simulink model "GS_s_v_seno_function"  (R2023b)
settings: Solver=VariableStepAuto  StartTime=0.0  StopTime=50  RelTol=1e-7
values from neighbouring files (symbols this model uses):
  omega_n = 2.63/Tr    (= 9.74074074074)    [gain_sheduling_WP5.m]
  zita = input(2)    [GS_compute_gains_PP.m]    (also in compute_gains_WP5.m; gain_sheduling_WP5.m = 0.95)
undefined symbols (not defined in the file or in its folder): LQR_activate
settings Model: Creator=miche  LastModifiedBy=miche

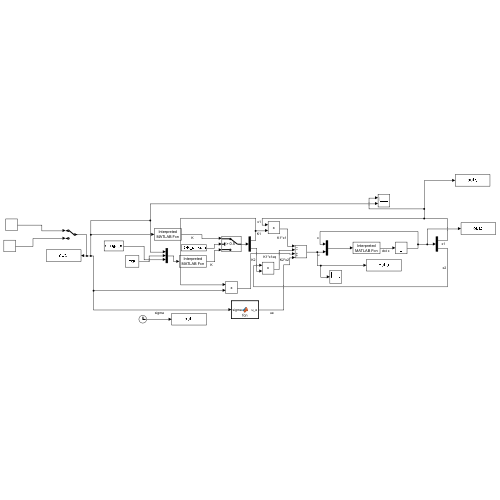
[thumbnail: Simulink's stored preview of the top-level diagram]
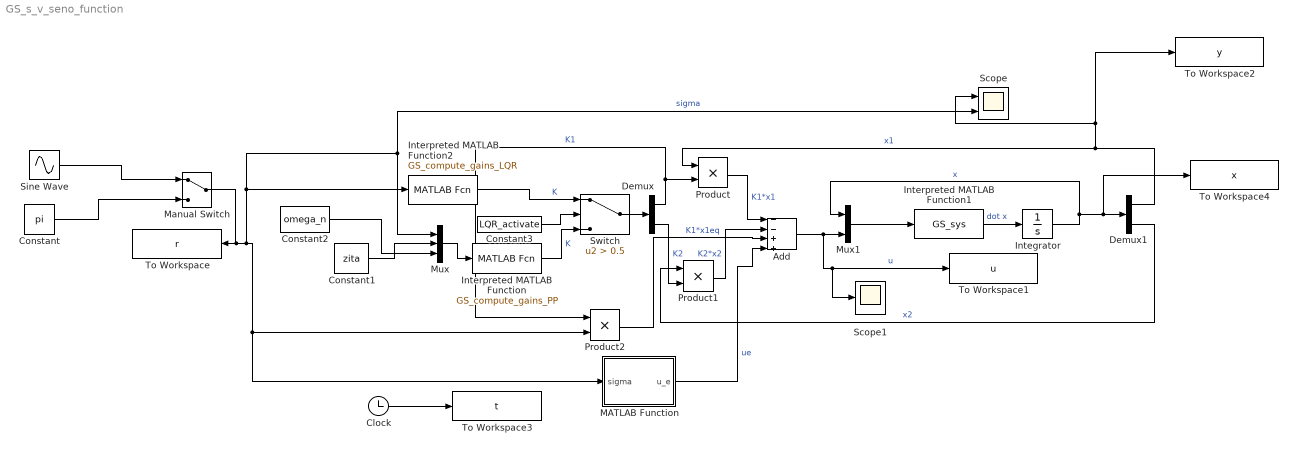
== system GS_s_v_seno_function ==
  Add : Sum  Inputs=--++
  Clock : Clock
  Constant : Constant  Value=pi
  Constant1 : Constant  Value=zita
  Constant2 : Constant  Value=omega_n
  Constant3 : Constant  Value=LQR_activate
  Demux : Demux  Outputs=2
  Demux1 : Demux  Outputs=2
  Integrator : Integrator
  Interpreted MATLAB Function : MATLABFcn  MATLABFcn=GS_compute_gains_PP  OutputDimensions=2
  Interpreted MATLAB Function1 : MATLABFcn  MATLABFcn=GS_sys  OutputDimensions=2
  Interpreted MATLAB Function2 : MATLABFcn  MATLABFcn=GS_compute_gains_LQR  OutputDimensions=2
  MATLAB Function : MATLAB Function  TreatAsAtomicUnit=on
  Manual Switch : ManualSwitch
  Mux : Mux  Inputs=3
  Mux1 : Mux  Inputs=2
  Product : Product
  Product1 : Product
  Product2 : Product
  Scope : Scope  NumInputPorts=2
  Scope1 : Scope
  Sine Wave : Sin  Amplitude=3.14  SampleTime=0
  Switch : Switch  Criteria=u2 > Threshold  Threshold=0.5  SaturateOnIntegerOverflow=off  InputSameDT=off
  To Workspace : ToWorkspace  VariableName=r  SampleTime=-1
  To Workspace1 : ToWorkspace  VariableName=u  SampleTime=-1
  To Workspace2 : ToWorkspace  VariableName=y  SampleTime=-1
  To Workspace3 : ToWorkspace  VariableName=t  SampleTime=-1
  To Workspace4 : ToWorkspace  VariableName=x  SampleTime=-1
  wires:
  Mux/1 -> Interpreted MATLAB Function/1
  Constant/1 -> Manual Switch/2
  Manual Switch/1 -> Scope/2, Mux/1, Interpreted MATLAB Function2/1, MATLAB Function/1(sigma), Product2/2, To Workspace/1  "sigma"
  Mux1/1 -> Interpreted MATLAB Function1/1
  Interpreted MATLAB Function1/1 -> Integrator/1  "dot x"
  Integrator/1 -> To Workspace4/1, Demux1/1, Mux1/1  "x"
  Product/1 -> Add/1  "K1*x1"
  Product1/1 -> Add/2  "K2*x2"
  Add/1 -> Scope1/1, To Workspace1/1, Mux1/2  "u"
  Demux/1 -> Product2/1, Product/2  "K1"
  Demux/2 -> Product1/2  "K2"
  Constant1/1 -> Mux/2
  Constant2/1 -> Mux/3
  Demux1/1 -> Product/1, To Workspace2/1, Scope/1  "x1"
  Sine Wave/1 -> Manual Switch/1
  Demux1/2 -> Product1/1  "x2"
  Product2/1 -> Add/3  "K1*x1eq"
  Clock/1 -> To Workspace3/1
  Switch/1 -> Demux/1
  Constant3/1 -> Switch/2
  Interpreted MATLAB Function/1 -> Switch/3  "K"
  Interpreted MATLAB Function2/1 -> Switch/1  "K"
  MATLAB Function/1(u_e) -> Add/4  "ue"

== matlab function GS_s_v_seno_function/MATLAB Function ==
  data: sigma input; u_e output
function u_e = fcn(sigma)

u_e=9.81*sin(sigma);
